simulink model "RM"  (R2013a)
settings: Solver=ode45  StartTime=0.0  StopTime=30.0  RelTol=1e-3
settings Model: Creator=Labo  LastModifiedBy=Labo

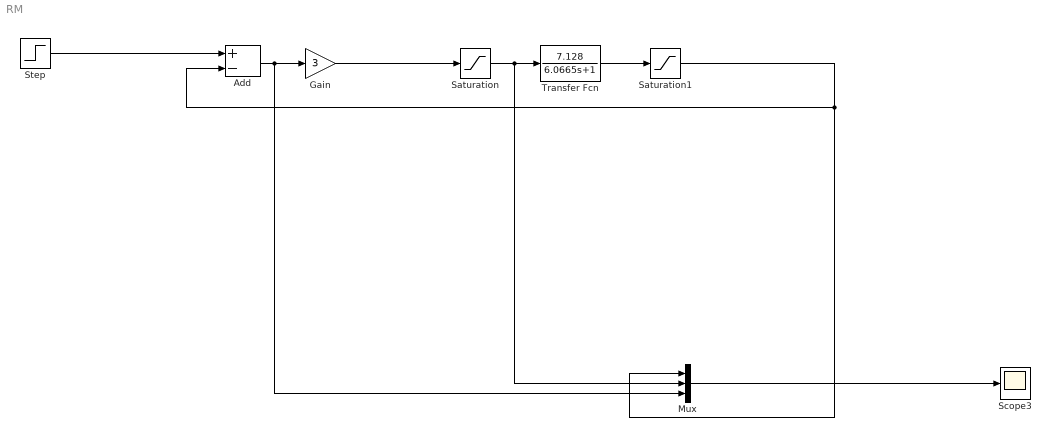
== system RM ==
  Add : Sum  Inputs=+-
  Gain : Gain  Gain=3
  Mux : Mux  Inputs=3
  Saturation : Saturate  UpperLimit=7.3  LowerLimit=-17.3
  Saturation1 : Saturate  UpperLimit=10-2.79  LowerLimit=-10-2.79
  Scope3 : Scope
  Step : Step  After=0.15  SampleTime=0
  Transfer Fcn : TransferFcn  Numerator=[7.128]  Denominator=[6.0665 1]  ContinuousStateAttributes='v'
  wires:
  Add/1 -> Gain/1, Mux/3
  Transfer Fcn/1 -> Saturation1/1
  Saturation1/1 -> Mux/1, Add/2
  Saturation/1 -> Mux/2, Transfer Fcn/1
  Mux/1 -> Scope3/1
  Step/1 -> Add/1
  Gain/1 -> Saturation/1
